simulink model "mass_sim"  (R2018a)
settings: Solver=ode45  StartTime=0.0  StopTime=P.t_end  RelTol=1e-3  EnableMultiTasking=on
InitFcn:
  | addpath ./..
  | mass_param
  | massParamHW7
undefined symbols (not defined in the file or in its folder): P
settings Model: Creator=beard  LastModifiedBy=mclain
settings DataIOCC: LimitDataPoints=on  SaveFormat=Array  SignalLoggingSaveFormat=ModelDataLogs
settings OptimizationCC: ExpressionDepthLimit=2147483647  InitFltsAndDblsToZero=on  LifeSpan=inf
settings DebuggingCC: UnderspecifiedInitializationDetection=Classic  MergeDetectMultiDrivingBlocksExec=none  SolverPrmCheckMsg=warning  FcnCallInpInsideContextMsg=warning  StateNameClashWarn=warning  SFUnexpectedBacktrackingDiag=warning  SFNoUnconditionalDefaultTransitionDiag=warning  SFExecutionAtInitializationDiag=none
settings HardwareCC: ProdBitPerPointer=32  ProdBitPerSizeT=32  ProdBitPerPtrDiffT=32  ProdLargestAtomicFloat=None  ProdIntDivRoundTo=Undefined  ProdEndianess=Unspecified  ProdWordSize=32  ProdHWDeviceType=32-bit Generic
settings ModelReferenceCC: PropagateSignalLabelsOutOfModel=off
settings CodeAppCC: StateflowObjectComments=on
settings GRTTargetCC: TargetLangStandard=C89/C90 (ANSI)  GeneratePreprocessorConditionals=Disable all  CombineOutputUpdateFcns=off  GRTInterface=on
settings ConfigComp: CovMetricSettings=dw  CovHtmlReporting=on  CovSaveCumulativeToWorkspaceVar=on  CovSaveSingleToWorkspaceVar=on  CovExternalEMLEnable=off

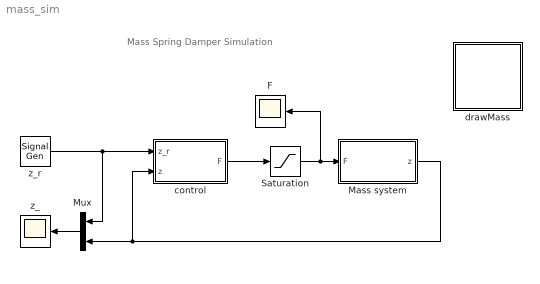
== system mass_sim ==
  note: Mass Spring Damper Simulation
  F : Scope
  Mass system : Subsystem
  Mux : Mux  Inputs=2
  Saturation : Saturate  UpperLimit=P.F_max  LowerLimit=-P.F_max
  control : Subsystem
  drawMass : Subsystem
      mask Display: image(imread('tv.jpg'))
  z_ : Scope
  z_r : SignalGenerator  WaveForm=square  Frequency=.02
  wires:
  Mux/1 -> z_/1
  z_r/1 -> Mux/1, control/1(z_r)
  control/1(F) -> Saturation/1
  Mass system/1(z) -> control/2(z), Mux/2
  Saturation/1 -> Mass system/1(F), F/1

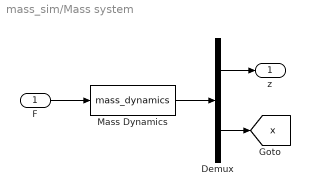
== system mass_sim/Mass system ==
  F : Inport
  Demux : Demux  Outputs=[1;2]
  Mass Dynamics : S-Function  FunctionName=mass_dynamics  Parameters=P  SFunctionDeploymentMode=off  EnableBusSupport=off
  z : Outport
  tag scope: x=global
  wires:
  F/1 -> Mass Dynamics/1
  Mass Dynamics/1 -> Demux/1
  Demux/1 -> z/1
  Demux/2 -> [x]

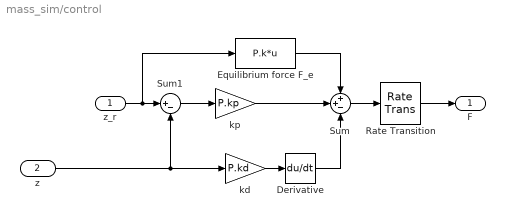
== system mass_sim/control ==
  z_r : Inport
  z : Inport  Port=2
  Derivative : Derivative  CoefficientInTFapproximation=P.sigma
  Equilibrium force F_e : Fcn  Expr=P.k*u
  Rate Transition : RateTransition  OutPortSampleTime=P.Ts
  Sum : Sum  Inputs=++-
  Sum1 : Sum  Inputs=|+-
  kd : Gain  Gain=P.kd
  kp : Gain  Gain=P.kp
  F : Outport
  wires:
  z/1 -> kd/1, Sum1/2
  z_r/1 -> Equilibrium force F_e/1, Sum1/1
  kd/1 -> Derivative/1
  Sum1/1 -> kp/1
  Derivative/1 -> Sum/3
  kp/1 -> Sum/2
  Equilibrium force F_e/1 -> Sum/1
  Rate Transition/1 -> F/1
  Sum/1 -> Rate Transition/1

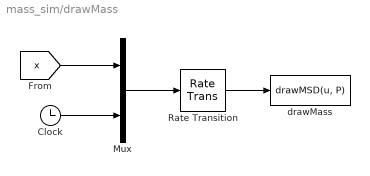
== system mass_sim/drawMass ==
  Clock : Clock
  Mux : Mux  Inputs=2
  Rate Transition : RateTransition  OutPortSampleTime=P.t_plot
  drawMass : MATLABFcn  MATLABFcn=drawMSD(u, P)  OutputDimensions=0
  wires:
  Mux/1 -> Rate Transition/1
  [x] -> Mux/1
  Clock/1 -> Mux/2
  Rate Transition/1 -> drawMass/1
